simulink model "Test_Multiplexer"  (Simulink 8.1)
settings: Solver=ode45  StartTime=0.0  StopTime=10.0  RelTol=1e-3
libraries: commutil2 x8, Byte_Multiplexers_Lib x4
settings Model: Creator=N  LastModifiedBy=uzivatel
settings DataIOCC: LimitDataPoints=off  SignalLoggingSaveFormat=Dataset
settings OptimizationCC: ExpressionDepthLimit=128
settings DebuggingCC: UnderspecifiedInitializationDetection=Simplified  MergeDetectMultiDrivingBlocksExec=error  SolverPrmCheckMsg=none  FcnCallInpInsideContextMsg=EnableAllAsError  FrameProcessingCompatibilityMsg=error  StateNameClashWarn=none
settings HardwareCC: ProdBitPerPointer=64  ProdLargestAtomicFloat=Float  ProdIntDivRoundTo=Zero  ProdEndianess=LittleEndian  ProdHWDeviceType=Intel->x86-64 (Windows64)
settings ModelReferenceCC: PropagateSignalLabelsOutOfModel=on
settings GRTTargetCC: CodeReplacementLibrary=None  CombineOutputUpdateFcns=on  CPPClassGenCompliant=on  GRTInterface=off

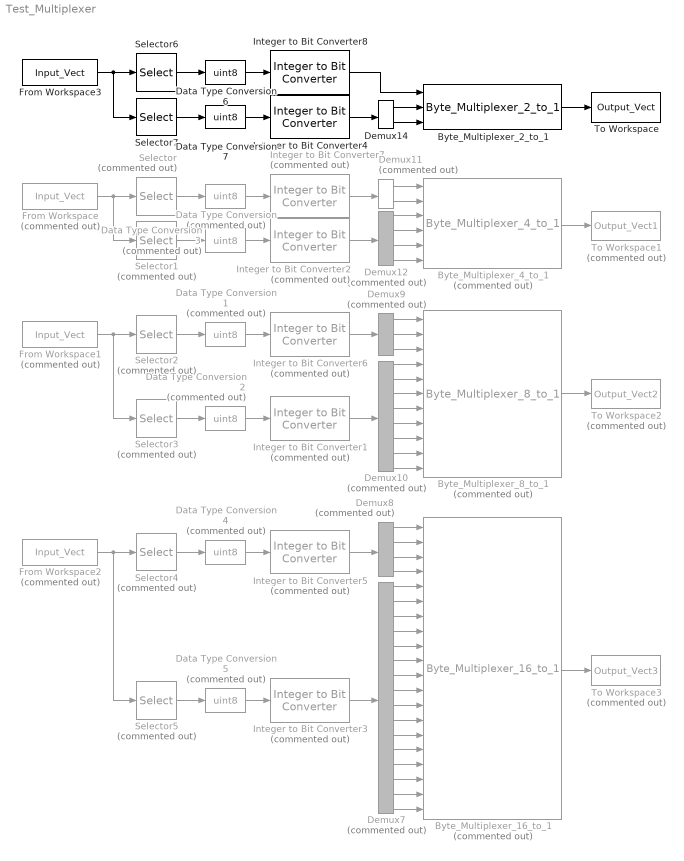
== system Test_Multiplexer ==
  Byte_Multiplexer_16_to_1 : Byte_Multiplexers_Lib/Byte_Multiplexers_Lib/Byte_Multiplexer_16_to_1  Commented=on
  Byte_Multiplexer_2_to_1 : Byte_Multiplexers_Lib/Byte_Multiplexers_Lib/Byte_Multiplexer_2_to_1
  Byte_Multiplexer_4_to_1 : Byte_Multiplexers_Lib/Byte_Multiplexers_Lib/Byte_Multiplexer_4_to_1  Commented=on
  Byte_Multiplexer_8_to_1 : Byte_Multiplexers_Lib/Byte_Multiplexers_Lib/Byte_Multiplexer_8_to_1  Commented=on
  Data Type Conversion{,1..5} (6 alike) : DataTypeConversion  Commented=on  OutDataTypeStr=uint8
  Data Type Conversion6 : DataTypeConversion  OutDataTypeStr=uint8
  Data Type Conversion7 : DataTypeConversion  OutDataTypeStr=uint8
  Demux10 : Demux  Commented=on  Outputs=8
  Demux11 : Demux  Commented=on  Outputs=2
  Demux12 : Demux  Commented=on
  Demux14 : Demux  Outputs=2
  Demux7 : Demux  Commented=on  Outputs=16
  Demux8 : Demux  Commented=on
  Demux9 : Demux  Commented=on  Outputs=3
  From Workspace : FromWorkspace  Commented=on  VariableName=Input_Vect  SampleTime=1  Interpolate=off  OutputAfterFinalValue=Holding final value
  From Workspace1 : FromWorkspace  Commented=on  VariableName=Input_Vect  SampleTime=1  Interpolate=off  OutputAfterFinalValue=Holding final value
  From Workspace2 : FromWorkspace  Commented=on  VariableName=Input_Vect  SampleTime=1  Interpolate=off  OutputAfterFinalValue=Holding final value
  From Workspace3 : FromWorkspace  VariableName=Input_Vect  SampleTime=1  Interpolate=off  OutputAfterFinalValue=Holding final value
  Integer to Bit Converter1 : commutil2/Integer to Bit Converter  Commented=on  nbits=8  signedInputValues=Unsigned  bitOrder=MSB first  outDtype=uint8
  Integer to Bit Converter2 : commutil2/Integer to Bit Converter  Commented=on  nbits=4  signedInputValues=Unsigned  bitOrder=MSB first  outDtype=uint8
  Integer to Bit Converter3 : commutil2/Integer to Bit Converter  Commented=on  nbits=16  signedInputValues=Unsigned  bitOrder=MSB first  outDtype=uint8
  Integer to Bit Converter4 : commutil2/Integer to Bit Converter  nbits=2  signedInputValues=Unsigned  bitOrder=MSB first  outDtype=uint8
  Integer to Bit Converter5 : commutil2/Integer to Bit Converter  Commented=on  nbits=4  signedInputValues=Unsigned  bitOrder=MSB first  outDtype=boolean
  Integer to Bit Converter6 : commutil2/Integer to Bit Converter  Commented=on  nbits=3  signedInputValues=Unsigned  bitOrder=MSB first  outDtype=boolean
  Integer to Bit Converter7 : commutil2/Integer to Bit Converter  Commented=on  nbits=2  signedInputValues=Unsigned  bitOrder=MSB first  outDtype=boolean
  Integer to Bit Converter8 : commutil2/Integer to Bit Converter  nbits=1  signedInputValues=Unsigned  bitOrder=MSB first  outDtype=boolean
  Selector : Selector  Commented=on  IndexMode=Zero-based  InputPortWidth=2  SampleTime=1  IndexOptions=Index vector (dialog)  Indices=0  OutputSizes=1
  Selector1 : Selector  Commented=on  IndexMode=Zero-based  InputPortWidth=2  IndexOptions=Index vector (dialog)  Indices=1  OutputSizes=1
  Selector2 : Selector  Commented=on  IndexMode=Zero-based  InputPortWidth=2  SampleTime=1  IndexOptions=Index vector (dialog)  Indices=0  OutputSizes=1
  Selector3 : Selector  Commented=on  IndexMode=Zero-based  InputPortWidth=2  IndexOptions=Index vector (dialog)  Indices=1  OutputSizes=1
  Selector4 : Selector  Commented=on  IndexMode=Zero-based  InputPortWidth=2  SampleTime=1  IndexOptions=Index vector (dialog)  Indices=0  OutputSizes=1
  Selector5 : Selector  Commented=on  IndexMode=Zero-based  InputPortWidth=2  IndexOptions=Index vector (dialog)  Indices=1  OutputSizes=1
  Selector6 : Selector  IndexMode=Zero-based  InputPortWidth=2  SampleTime=1  IndexOptions=Index vector (dialog)  Indices=0  OutputSizes=1
  Selector7 : Selector  IndexMode=Zero-based  InputPortWidth=2  IndexOptions=Index vector (dialog)  Indices=1  OutputSizes=1
  To Workspace : ToWorkspace  VariableName=Output_Vect  SampleTime=1
  To Workspace1 : ToWorkspace  Commented=on  VariableName=Output_Vect1  SampleTime=1
  To Workspace2 : ToWorkspace  Commented=on  VariableName=Output_Vect2  SampleTime=1
  To Workspace3 : ToWorkspace  Commented=on  VariableName=Output_Vect3  SampleTime=1
  wires:
  Integer to Bit Converter5/1 -> Demux8/1
  Integer to Bit Converter3/1 -> Demux7/1
  Demux7/1 -> Byte_Multiplexer_16_to_1/5
  Byte_Multiplexer_16_to_1/1 -> To Workspace3/1
  Demux7/2 -> Byte_Multiplexer_16_to_1/6
  Demux7/3 -> Byte_Multiplexer_16_to_1/7
  Demux7/4 -> Byte_Multiplexer_16_to_1/8
  Demux7/5 -> Byte_Multiplexer_16_to_1/9
  Demux7/6 -> Byte_Multiplexer_16_to_1/10
  Demux7/7 -> Byte_Multiplexer_16_to_1/11
  Demux7/8 -> Byte_Multiplexer_16_to_1/12
  Demux7/9 -> Byte_Multiplexer_16_to_1/13
  Demux7/10 -> Byte_Multiplexer_16_to_1/14
  Demux7/11 -> Byte_Multiplexer_16_to_1/15
  Demux7/12 -> Byte_Multiplexer_16_to_1/16
  Demux7/13 -> Byte_Multiplexer_16_to_1/17
  Demux7/14 -> Byte_Multiplexer_16_to_1/18
  Demux7/15 -> Byte_Multiplexer_16_to_1/19
  Demux7/16 -> Byte_Multiplexer_16_to_1/20
  Demux8/1 -> Byte_Multiplexer_16_to_1/1
  Demux8/3 -> Byte_Multiplexer_16_to_1/3
  Demux8/2 -> Byte_Multiplexer_16_to_1/2
  Demux8/4 -> Byte_Multiplexer_16_to_1/4
  Byte_Multiplexer_4_to_1/1 -> To Workspace1/1
  Byte_Multiplexer_8_to_1/1 -> To Workspace2/1
  Demux9/1 -> Byte_Multiplexer_8_to_1/1
  Demux9/2 -> Byte_Multiplexer_8_to_1/2
  Demux9/3 -> Byte_Multiplexer_8_to_1/3
  Integer to Bit Converter6/1 -> Demux9/1
  Demux10/1 -> Byte_Multiplexer_8_to_1/4
  Demux10/2 -> Byte_Multiplexer_8_to_1/5
  Demux10/3 -> Byte_Multiplexer_8_to_1/6
  Demux10/4 -> Byte_Multiplexer_8_to_1/7
  Demux10/5 -> Byte_Multiplexer_8_to_1/8
  Demux10/6 -> Byte_Multiplexer_8_to_1/9
  Demux10/7 -> Byte_Multiplexer_8_to_1/10
  Demux10/8 -> Byte_Multiplexer_8_to_1/11
  Demux11/2 -> Byte_Multiplexer_4_to_1/2
  Integer to Bit Converter7/1 -> Demux11/1
  Demux12/1 -> Byte_Multiplexer_4_to_1/3
  Demux12/2 -> Byte_Multiplexer_4_to_1/4
  Demux12/3 -> Byte_Multiplexer_4_to_1/5
  Demux12/4 -> Byte_Multiplexer_4_to_1/6
  Demux11/1 -> Byte_Multiplexer_4_to_1/1
  Demux14/1 -> Byte_Multiplexer_2_to_1/2
  Demux14/2 -> Byte_Multiplexer_2_to_1/3
  From Workspace/1 -> Selector1/1, Selector/1
  Selector/1 -> Data Type Conversion/1
  Selector1/1 -> Data Type Conversion3/1
  Data Type Conversion3/1 -> Integer to Bit Converter2/1
  Byte_Multiplexer_2_to_1/1 -> To Workspace/1
  From Workspace1/1 -> Selector3/1, Selector2/1
  Selector2/1 -> Data Type Conversion1/1
  Selector3/1 -> Data Type Conversion2/1
  Data Type Conversion1/1 -> Integer to Bit Converter6/1
  Data Type Conversion2/1 -> Integer to Bit Converter1/1
  From Workspace2/1 -> Selector5/1, Selector4/1
  Selector4/1 -> Data Type Conversion4/1
  Selector5/1 -> Data Type Conversion5/1
  Data Type Conversion4/1 -> Integer to Bit Converter5/1
  Data Type Conversion5/1 -> Integer to Bit Converter3/1
  Integer to Bit Converter1/1 -> Demux10/1
  Integer to Bit Converter2/1 -> Demux12/1
  Data Type Conversion/1 -> Integer to Bit Converter7/1
  Integer to Bit Converter8/1 -> Byte_Multiplexer_2_to_1/1
  From Workspace3/1 -> Selector7/1, Selector6/1
  Selector6/1 -> Data Type Conversion6/1
  Selector7/1 -> Data Type Conversion7/1
  Data Type Conversion7/1 -> Integer to Bit Converter4/1
  Integer to Bit Converter4/1 -> Demux14/1
  Data Type Conversion6/1 -> Integer to Bit Converter8/1
